simulink library "Cust_Library_planarPKM"  (R2024a)
settings: Solver=VariableStepAuto  StartTime=0.0  StopTime=10.0  RelTol=1e-3
undefined symbols (not defined in the file): param
libraries: simulink x1
(part 2 of 2)

== matlab function Cust_Library_planarPKM/Calculate time derivatives of Jacobian/Calculate_derivative_of_Jacobian_matrices ==
  data: qj_rad input; xEE_ input; dqj_rad input; dxEE_ input; dJinv_hredqax_3RRRreturn output; dJ_hredxqa_3RRRreturn output; dJinv_hqx_3RRRreturn output; l_all parameter; dJacA_hredx_3RRRreturn output; dJacB_hredqa_3RRRreturn output; r_BasisPla_MobPla parameter
function [dJinv_hredqax_3RRRreturn, dJ_hredxqa_3RRRreturn, dJinv_hqx_3RRRreturn, dJacA_hredx_3RRRreturn, dJacB_hredqa_3RRRreturn] ...
    = calcJac(qj_rad, xEE_, dqj_rad, dxEE_, l_all, r_BasisPla_MobPla)
    % Function for determining the time derivatives of the Jacobi matrices based on complete constraints h and reduced constraints hred  
    % Input:
    % qj_rad in rad: Joint coordinates (9x1)
    % dqj_rad in rad: Joint velocities (9x1)
    % xEE_ in m and rad: Platform coordinates in the base CS (3x1)
    % dxEE_ in m and rad: Platform velocities (3x1)
    %
    % Output:
    % dJinv_hqx_3RRRreturn: Time derivative of the Jacobian matrix for projection from ddx to ddq(3x9)
    % dJ_hredxqa_3RRreturn: Temporal derivative of the Jacobian matrix for projection ddqa onto ddx (3x3)
    % dJinv_hredqax_3RRreturn: Temporal derivative of the Jacobian matrix for projection ddx onto ddqa (3x3)
    
    % Aran Mohammad, aran.mohammad@imes.uni-hannover.de, 2022-12
    % (C) Institute for Mechatronic Systems, Leibniz University Hanover
      
      
xEE = [xEE_(1); xEE_(2); 0; 0; 0; xEE_(3)];
dxEE = [dxEE_(1); dxEE_(2); 0; 0; 0; dxEE_(3)];


dJinv_hredqax_3RRRreturn = dJinv_hredqax_3RRR(qj_rad, dqj_rad, xEE, dxEE, l_all, r_BasisPla_MobPla);

dJ_hredxqa_3RRRreturn = dJ_hredxqa_3RRR(qj_rad, dqj_rad, xEE, dxEE, l_all, r_BasisPla_MobPla);

dJinv_hqx_3RRRreturn = transpose(dJinv_hqx_3RRR(qj_rad, dqj_rad, xEE, dxEE, l_all, r_BasisPla_MobPla));

dJacA_hredx_3RRRreturn = dJacA_hredx_3RRR(qj_rad, dqj_rad, xEE, dxEE, l_all, r_BasisPla_MobPla);
dJacB_hredqa_3RRRreturn = dJacB_hredqa_3RRR(qj_rad, dqj_rad, xEE, dxEE, l_all, r_BasisPla_MobPla);

== matlab function Cust_Library_planarPKM/Calculate Jacobian matrices/calculate_Jacobian ==
  data: qj_rad input; xEE_ input; det_JacA_hredx_3RRR output; det_JacB_hredqa_3RRR output; cond_JacA_hredx_3RRR output; cond_JacB_hredqa_3RRR output; JacA_hredx_3RRR output; JacB_hredqa_3RRR output; J_hredxqa_ind_3RRRreturn output; Jinv_hredqax_ind_3RRRreturn output; Jinv_hqx_ind_3RRRreturn output; l_all_id parameter; det_JacA_hredx_ind_3RRRreturn_homogen output; det_JacB_hredqa_ind_3RRRreturn_homogen output; Jinv_hqx_dq_dqa output; cond_Jac_hredxqa_3RRR output; r_fixPlat_j parameter; r_mobPlat_j parameter; beta_j parameter; psi_j parameter
function [det_JacA_hredx_3RRR, det_JacB_hredqa_3RRR, cond_JacA_hredx_3RRR, cond_JacB_hredqa_3RRR, ...
          JacA_hredx_3RRR, JacB_hredqa_3RRR, J_hredxqa_ind_3RRRreturn, Jinv_hredqax_ind_3RRRreturn,...
          Jinv_hqx_ind_3RRRreturn, det_JacA_hredx_ind_3RRRreturn_homogen, det_JacB_hredqa_ind_3RRRreturn_homogen, ...
          Jinv_hqx_dq_dqa, cond_Jac_hredxqa_3RRR] = calcJac(qj_rad, xEE_, l_all_id, r_fixPlat_j, r_mobPlat_j, beta_j, psi_j)
    % Function for determining the Jacobi matrices based on complete constraints h and reduced constraints hred  
    % Input:
    % qj_rad in rad: Joint coordinates (9x1)
    % xEE_ in m and rad: Platform coordinates in the base CS (3x1)
    %
    % Output:
    % JacA_hredx_ind_3RRRreturn: Jacobian matrix of the direct kinematics (3x3)
    % JacB_hredqa_ind_3RRreturn: Jacobian matrix of the inverse kinematics (3x3)
    % Jinv_hqx_ind_3RRreturn: Inverse Jacobian matrix for projection from dx to dq(3x9)
    % J_hredxqa_ind_3RRreturn: Jacobian matrix for projection dqa onto dx (3x3)
    % Jinv_hredqax_ind_3RRreturn: Inverse Jacobian matrix for projection dx onto dqa (3x3)
    % det_JacA_hredx_3RRR: Determinant of the Jacobian matrix of the direct kinematics (1x1)
    % det_JacB_hredqa_3RRR: Determinant of the Jacobian matrix of the inverse kinematics (1x1)
   
    % Aran Mohammad, aran.mohammad@imes.uni-hannover.de, 2022-12
    % (C) Institute for Mechatronic Systems, Leibniz University Hanover
      
xEE = [xEE_(1); xEE_(2); 0; 0; 0; xEE_(3)];

Jinv_hqx_3RRRreturn = zeros(3,3);%transpose(Jinv_hqx_3RRR(qj_rad, xEE, l_all, r_BasisPla_MobPla));
Jinv_hredqax_3RRRreturn = zeros(3,3);%Jinv_hredqax_3RRR(qj_rad, xEE, l_all, r_BasisPla_MobPla);
J_hredxqa_3RRRreturn = zeros(3,3);% J_hredxqa_3RRR(qj_rad, xEE, l_all, r_BasisPla_MobPla);

%% individuelle kinematische Parameter
JacA_hredx_ind_3RRRreturn = JacA_hredx_ind_3RRR(qj_rad, xEE, l_all_id, r_fixPlat_j, r_mobPlat_j, psi_j, beta_j);
JacB_hredqa_ind_3RRRreturn = JacB_hredqa_ind_3RRR(qj_rad, xEE, l_all_id, r_fixPlat_j, r_mobPlat_j, psi_j, beta_j);
Jinv_hqx_ind_3RRRreturn = transpose(Jinv_hqx_ind_3RRR(qj_rad, xEE, l_all_id, r_fixPlat_j, r_mobPlat_j, psi_j, beta_j));

Jinv_hredqax_ind_3RRRreturn = -inv(JacB_hredqa_ind_3RRRreturn)*JacA_hredx_ind_3RRRreturn;
J_hredxqa_ind_3RRRreturn = inv(Jinv_hredqax_ind_3RRRreturn);

Jinv_hqx_dq_dqa = Jinv_hqx_ind_3RRRreturn / Jinv_hredqax_ind_3RRRreturn;

JacA_hredx_3RRR = JacA_hredx_ind_3RRRreturn;
JacB_hredqa_3RRR = JacB_hredqa_ind_3RRRreturn;

% Determinanten
det_JacA_hredx_3RRR = det(JacA_hredx_ind_3RRRreturn);
det_JacB_hredqa_3RRR = det(JacB_hredqa_ind_3RRRreturn);
cond_JacA_hredx_3RRR = cond(JacA_hredx_ind_3RRRreturn,2);
cond_JacB_hredqa_3RRR = cond(JacB_hredqa_ind_3RRRreturn,2);
cond_Jac_hredxqa_3RRR = cond(J_hredxqa_ind_3RRRreturn,2);


JacA_hredx_ind_3RRRreturn_homogen = JacA_hredx_ind_3RRRreturn;
JacA_hredx_ind_3RRRreturn_homogen(:,3) = JacA_hredx_ind_3RRRreturn(:,3)./r_mobPlat_j(1);
JacB_hredqa_ind_3RRRreturn_homogen = JacB_hredqa_ind_3RRRreturn./l_all_id(1);
det_JacA_hredx_ind_3RRRreturn_homogen = det(JacA_hredx_ind_3RRRreturn_homogen);
det_JacB_hredqa_ind_3RRRreturn_homogen = det(JacB_hredqa_ind_3RRRreturn_homogen);

== matlab function Cust_Library_planarPKM/Localize contact point on second link via particle filter/MATLAB Function4 ==
  data: trigger input; Tauext input; predLoc_2D output; predBody input; q input; dq input; x input; dx input; Jinv_hqx_ind input; J_hredxqa input; n_particle input; predForce_2D output; l_all parameter; predLoc_3D output; predForce_3D output; r_BasisPla_MobPla parameter; l_all_id parameter; r_fixPlat_j parameter; r_mobPlat_j parameter; psi_j parameter; x_N_2D parameter; x_CovR_Inv_2D parameter; x_N_3D parameter; x_CovR_Inv_3D parameter; pf_dim parameter
function [predLoc_2D, predForce_2D, predLoc_3D, predForce_3D] = ...
    LocIsol_particleFilter_red_(trigger, Tauext,predBody, q, dq, x, dx, Jinv_hqx_ind, J_hredxqa,...
    n_particle, l_all, r_BasisPla_MobPla, l_all_id, r_fixPlat_j, r_mobPlat_j, psi_j, x_N_2D, x_CovR_Inv_2D, x_N_3D, x_CovR_Inv_3D, pf_dim)
   
    predLoc_2D = 0;
    predForce_2D = 0;
    predLoc_3D = 0;
    predForce_3D = zeros(1,2);
    if pf_dim == 2
        [predLoc_2D, predForce_2D, ~, ~] = LocIsol_particleFilter_red(trigger,Tauext, predBody, q, dq, x, dx, Jinv_hqx_ind, J_hredxqa, ...
            n_particle, l_all, r_BasisPla_MobPla, l_all_id, r_fixPlat_j, r_mobPlat_j, psi_j, x_N_2D, x_CovR_Inv_2D);
    elseif pf_dim == 3
        [predLoc_3D, predForce_3D, ~, ~] = LocIsol_particleFilter(trigger, Tauext, predBody, q, dq, x, dx, Jinv_hqx_ind, J_hredxqa,...
            n_particle, l_all, r_BasisPla_MobPla, l_all_id, r_fixPlat_j, r_mobPlat_j, psi_j, x_N_3D, x_CovR_Inv_3D);
    end
end

== matlab function Cust_Library_planarPKM/Moe_ArMo ==
  data: x_soll input; mode output size=1; x_ist input; qa_ist input; dqa_ist input; dx_soll input; J_hredxqa input; ddx_soll input; dJ_hredxqa input; param parameter; tau_soll output size=[3,1]; MMQa_ist input; dx_ist input; ddqa_prev input; dqa_out output; ddqa_out output; tau_out output; e_qa output size=[3,1]; de_qa output size=[3,1]; qa_soll output size=[3,1]; dqa_prev input size=[3,1]; h_kappa_out output size=1; dq_all output size=[12,1]; ddq_all output size=[12,1]; tau_all output size=[12,1]; mode_prev input; D_pose input; K_pose input; tau_prev input; taucX_ist input; kappa_ist input; min_dist input; sigma_activ_list output; h_kappa_flag_out output; x_soll_r output; dkappa input; dmindist input; J_kappa input; J_dist input; dJ_kappa input; dJ_dist input; MMX_ist input; taucQa_ist input; tauCQa_ist input; xp_soll input; dxp_soll input; ddxp_soll input; xp_KSGj_ist input; dxp_KSGj_ist input; dRxp_ist input; R_0Gj input; dR_0Gj input; J_xpqa input; J_xpqa_KS0 input; dJ_xpqa_KS0 input; dxp_KS0_ist input; xp_KS0_ist input; dJ_xpqa input; predbody input; BP_Retr_calc_run_KSGj input; rr_level input; rueck_KS0 input; lambda_dq input; lambda_ddq input; lambda_tau input; pd_reglerQ input; kappa_mindist_lim input; priority_x input; gain_check_status_kappa input; gain_check_status_mindist input; activate_bp_UNB input; kappa_traj_soll input; mindist_traj_soll input; rueckzug_aktiv input; reaction_angle_rad input; x_ist_r output; dq_Jkappa output; dq_Jdist output; mode_nan output; clamping_predicted input; clampingBody_predicted input; clampingreaction_aktiv input; traj_qap_soll_cl input; J_q_qa input; dJ_q_qa input; M_kappa output; M_dist output; q_ist_rad input; dq_ist_rads input
function [mode, tau_soll, dqa_out, ddqa_out, tau_out, e_qa, de_qa, qa_soll,...
          h_kappa_out, dq_all,  ddq_all, tau_all, sigma_activ_list, h_kappa_flag_out, ...
          x_soll_r, x_ist_r, dq_Jkappa, dq_Jdist, mode_nan, M_kappa, M_dist] = ...
            fcn(x_soll, x_ist, qa_ist, dqa_ist, dx_soll, J_hredxqa, ddx_soll, ...
                dJ_hredxqa, param, MMQa_ist, dx_ist, ddqa_prev, dqa_prev, mode_prev, ...
                D_pose, K_pose, tau_prev, taucX_ist, kappa_ist, min_dist, dkappa, ...
                dmindist, J_kappa, J_dist, dJ_kappa, dJ_dist, MMX_ist, taucQa_ist, ...
                tauCQa_ist, xp_soll, dxp_soll, ddxp_soll, xp_KSGj_ist, dxp_KSGj_ist, dRxp_ist, ...
                R_0Gj, dR_0Gj, J_xpqa, J_xpqa_KS0, dJ_xpqa_KS0, dxp_KS0_ist, xp_KS0_ist, ...
                dJ_xpqa, predbody, BP_Retr_calc_run_KSGj, rr_level, rueck_KS0, ...
                lambda_dq, lambda_ddq, lambda_tau, pd_reglerQ, kappa_mindist_lim, priority_x,   gain_check_status_kappa, gain_check_status_mindist,...
                activate_bp_UNB, kappa_traj_soll, mindist_traj_soll, rueckzug_aktiv, reaction_angle_rad,...
                clamping_predicted, clampingBody_predicted, clampingreaction_aktiv, traj_qap_soll_cl, J_q_qa, dJ_q_qa, q_ist_rad, dq_ist_rads)
            

       mode = zeros(1,1);
       tau_soll = zeros(3,1);
       dqa_out = zeros(3,1);
       ddqa_out = zeros(3,1);
       tau_out = zeros(3,1);
       e_qa = zeros(3,1);
       de_qa = zeros(3,1);
       qa_soll = zeros(3,1);
       h_kappa_out = zeros(1,1);
       dq_all = zeros(12,1);
       ddq_all = zeros(12,1);
       tau_all = zeros(12,1);
       sigma_activ_list = zeros(8,1);
       h_kappa_flag_out = zeros(1,1);
       x_soll_r = zeros(3,1);
       x_ist_r = zeros(3,1);
       dq_Jkappa = zeros(4,1);
       dq_Jdist  = zeros(4,1);
       mode_nan = 0;
       M_kappa = nan;
       M_dist = nan;
    if rr_level ~= 0 %&& rueckzug_aktiv
        [mode, tau_soll, dqa_out, ddqa_out, tau_out, e_qa, de_qa, qa_soll,...
          h_kappa_out, dq_all,  ddq_all, tau_all, sigma_activ_list, h_kappa_flag_out, ...
          x_soll_r, x_ist_r, dq_Jkappa, dq_Jdist, mode_nan, M_kappa, M_dist] = ...
        calc_rr(x_soll, x_ist, qa_ist, dqa_ist, dx_soll, J_hredxqa, ddx_soll, ...
                    dJ_hredxqa, param, MMQa_ist, dx_ist, ddqa_prev, dqa_prev, mode_prev, ...
                    D_pose, K_pose, tau_prev, taucX_ist, kappa_ist, min_dist, dkappa, ...
                    dmindist, J_kappa, J_dist, dJ_kappa, dJ_dist, MMX_ist, taucQa_ist, ...
                    tauCQa_ist, xp_soll, dxp_soll, ddxp_soll, xp_KSGj_ist, dxp_KSGj_ist, dRxp_ist, ...
                    R_0Gj, dR_0Gj, J_xpqa, J_xpqa_KS0, dJ_xpqa_KS0, dxp_KS0_ist, xp_KS0_ist, ...
                    dJ_xpqa, predbody, BP_Retr_calc_run_KSGj, rr_level, rueck_KS0, ...
                    lambda_dq, lambda_ddq, lambda_tau, pd_reglerQ, kappa_mindist_lim, priority_x,   gain_check_status_kappa, gain_check_status_mindist,...
                    activate_bp_UNB, kappa_traj_soll, mindist_traj_soll, rueckzug_aktiv, reaction_angle_rad,...
                    clamping_predicted, clampingBody_predicted, clampingreaction_aktiv, traj_qap_soll_cl, J_q_qa, dJ_q_qa, q_ist_rad, dq_ist_rads);

    else 
       mode = zeros(1,1);
       tau_soll = zeros(3,1);
       dqa_out = zeros(3,1);
       ddqa_out = zeros(3,1);
       tau_out = zeros(3,1);
       e_qa = zeros(3,1);
       de_qa = zeros(3,1);
       qa_soll = zeros(3,1);
       h_kappa_out = zeros(1,1);
       dq_all = zeros(12,1);
       ddq_all = zeros(12,1);
       tau_all = zeros(12,1);
       sigma_activ_list = zeros(8,1);
       h_kappa_flag_out = zeros(1,1);
       x_soll_r = zeros(3,1);
       x_ist_r = zeros(3,1);
       dq_Jkappa = zeros(4,1);
       dq_Jdist  = zeros(4,1);
       mode_nan = 0;
       M_kappa = nan;
       M_dist = nan;
    end

== stateflow chart Cust_Library_planarPKM/Statemachine ==
  state State0 %Eingang, warte auf kommunikation mit den Motoren
    entry:
    control 		= 4;%Ist-Winkel in die BP
    bp_on 		= 0;%BP unbenutzt
    bp_retr_on       = 0;% BP für Retr unbenutzt
    tr_on 		      = 0;%Traj unbenutzt
    gmt_on            = 0;%GMT unbenutzt
    error 			= 0;%Motor kann starten
    control_out      = 0;%Ist-Werte als Soll-Werte
    state = 0;
  state State1 %Kommunikation funktioniert
    entry:
    control 		= 4;%Ist-Winkel in die BP
    bp_on 		= 0;%BP unbenutzt
    bp_retr_on       = 0;% BP für Retr unbenutzt
    tr_on 		      = 0;%Traj unbenutzt
    gmt_on            = 0;%GMT unbenutzt
    error 			= 0;%Motor kann starten
    control_out      = 0;%Ist-Werte als Soll-Werte
    state = 1;
  state Home Position Drive [group]
    state State7 %Setzte Vorgaben, Überprüfe ob
      %Zielpunkt valid ist
      entry:
      control 		 	= 2;%Home-Winkel in die BP
      bp_on 			= 0; %BP unbenutzt
      bp_retr_on       = 0;% BP für Retr unbenutzt
      tr_on 		      = 0;%Traj unbenutzt
      gmt_on            = 0;%GMT unbenutzt
      error 			= 0;%Motor bleibt an
      control_out      = 1;%BP-Werte als Soll-Werte
      state = 7;
    state State8 %Starte Bahnplanung
      entry:
      control 		 	= 2;%Ziel-Winkel in die BP
      bp_on 			= 1; %BP wird genutzt
      bp_retr_on       = 0;% BP für Retr unbenutzt
      tr_on 		      = 0;%Traj unbenutzt
      gmt_on            = 0;%GMT unbenutzt
      error 			= 0;%Motor bleibt an
      control_out      = 1;%BP-Werte als Soll-Werte
      state = 8;
    state State9 %Starte Bahnplanung
      entry:
      control 		 	= 2;%Ziel-Winkel in die BP
      bp_on 			= 0; %BP beendet
      bp_retr_on       = 0;% BP für Retr unbenutzt
      tr_on 		      = 0;%Traj unbenutzt
      gmt_on            = 0;%GMT unbenutzt
      error 			= 0;%Motor bleibt an
      control_out      = 1;%BP-Werte als Soll-Werte
      state = 9;
    State7 %Setzte Vorgaben, Überprüfe ob -> State8 %Starte Bahnplanung [order 1] : [bp_valid ==1]
    State8 %Starte Bahnplanung -> State9 %Starte Bahnplanung [order 2] : [bp_calc_run == 0]
  state Trajectory Drive [group]
    state State10 %Setzte Vorgaben, Überprüfe ob
      %Zielpunkt valid ist
      entry:
      control 		 	= 3;%Startwinkel der traj in BP
      bp_on 			= 0;%BP unbenutzt
      bp_retr_on       = 0;% BP für Retr unbenutzt
      tr_on 			= 0;%Traj unbenutzt
      gmt_on            = 0;%GMT unbenutzt
      error 			= 0;%Motor bleibt an
      control_out      = 1;%BP-Werte als Soll-Werte
      state = 10;
    state State11 %Fahre zum Ausgangspunkt
      entry:
      control 		 	= 3;%Startwinkel der traj in BP
      bp_on 			= 1;%BP wird genutzt
      bp_retr_on       = 0;% BP für Retr unbenutzt
      tr_on 			= 0;%Traj unbenutzt
      gmt_on            = 0;%GMT unbenutzt
      error 			= 0;%Motor bleibt an
      control_out      = 1;%BP-Werte als Soll-Werte
      state = 11;
    state State12 %Validiere Trajektorie und setze Vorgaben
      entry:
      control 		 	= 4;%Ist-Winkel in die BP
      bp_on 			= 0;%BP unbenutzt
      bp_retr_on       = 0;% BP für Retr unbenutzt
      tr_on 			= 0;%Traj unbenutzt
      gmt_on            = 0;%GMT unbenutzt
      error 			= 0;%Motor bleibt an
      control_out      = 1;%BP-Werte als Soll-Werte
      state = 12;
    state State13 %Starte Trajektorie
      entry:
      control 		 	= 4;%Ist-Winkel in die BP
      bp_on 			= 0;%BP unbenutzt
      bp_retr_on       = 0;% BP für Retr unbenutzt
      tr_on 		      = 1;%Traj wird genutzt
      gmt_on            = 0;%GMT unbenutzt
      error 			= 0;%Motor bleibt an
      control_out      = 2;%Traj-Werte als Soll-Werte
      state = 13;
    state State14 %Starte Trajektorie
      entry:
      control 		 	= 4;%Ist-Winkel in die BP
      bp_on 			= 0;%BP unbenutzt
      bp_retr_on       = 0;% BP für Retr unbenutzt
      tr_on 		      = 0;%Traj unbenutzt
      gmt_on            = 0;%GMT unbenutzt
      error 			= 0;%Motor bleibt an
      control_out      = 2;%Traj-Werte als Soll-Werte
      state = 14;
    State10 %Setzte Vorgaben, Überprüfe ob -> State11 %Fahre zum Ausgangspunkt [order 1] : [bp_valid ==1]
    State11 %Fahre zum Ausgangspunkt -> State12 %Validiere Trajektorie und setze Vorgaben [order 1] : [bp_calc_run ==0  & tr_in_starting_pos == 1]
    State12 %Validiere Trajektorie und setze Vorgaben -> State13 %Starte Trajektorie [order 1] : [tr_valid == 1]
    State13 %Starte Trajektorie -> State14 %Starte Trajektorie [order 2] : [tr_calc_run ==0]
  state Target Position Drive [group]
    state State2 %Setzte Vorgaben, Überprüfe ob
      %Zielpunkt valid ist
      entry:
      control 			= 1;%Ziel-Winkel in die BP
      bp_on 			= 0; %BP unbenutzt
      bp_retr_on       = 0;% BP für Retr unbenutzt
      tr_on 		      = 0;%Traj unbenutzt
      gmt_on            = 0;%GMT unbenutzt
      error 			= 0;%Motor bleibt an
      control_out      = 1;%BP-Werte als Soll-Werte
      state = 2;
    state State3 %Starte Bahnplanung
      entry:
      control 			= 1;%Ziel-Winkel in die BP
      bp_on 			= 1; %BP wird genutzt
      bp_retr_on       = 0;% BP für Retr unbenutzt
      tr_on 		      = 0;%Traj unbenutzt
      gmt_on            = 0;%GMT unbenutzt
      error 			= 0;%Motor bleibt an
      control_out      = 1;%BP-Werte als Soll-Werte
      state = 3;
    state State4 %Starte Bahnplanung
      entry:
      control 			= 1;%Ziel-Winkel in die BP
      bp_on 			= 0; %BP beendet
      bp_retr_on       = 0;% BP für Retr unbenutzt
      tr_on 		      = 0;%Traj unbenutzt
      gmt_on            = 0;%GMT unbenutzt
      error 			= 0;%Motor bleibt an
      control_out      = 1;%BP-Werte als Soll-Werte
      state = 4;
    State2 %Setzte Vorgaben, Überprüfe ob -> State3 %Starte Bahnplanung [order 1] : [bp_valid ==1]
    State3 %Starte Bahnplanung -> State4 %Starte Bahnplanung [order 1] : [bp_calc_run == 0]
  state Geomagic Touch [group]
    state State15
      entry:
      control 		 	= 2;%Startwinkel der traj in BP
      bp_on 			= 0;%BP unbenutzt
      bp_retr_on       = 0;% BP für Retr unbenutzt
      tr_on 			= 0;%Traj unbenutzt
      gmt_on            = 1;%GMT benutzt
      error 			= 0;%Motor bleibt an
      control_out      = 3;%GMT-Werte als Soll-Werte
      state = 15;
  state Retraction Drive [group]
    state State25 %Setzte Vorgaben, Überprüfe ob
      %Zielpunkt valid ist
      entry:
      control 			= 5;%Ziel-Winkel in die BP
      bp_on 			= 1; %BP unbenutzt
      bp_retr_on       = 0;% BP für Retr unbenutzt
      tr_on 		      = 0;%Traj unbenutzt
      gmt_on            = 0;%GMT unbenutzt
      error 			= 0;%Motor bleibt an
      control_out      = 1;%BP-Werte als Soll-Werte
      state = 25;
    state State26 %Starte Bahnplanung
      entry:
      control 			= 5;%Ziel-Winkel in die BP
      bp_on 			= 1; %BP unbenutzt
      bp_retr_on       = 1;% BP für Retr wird benutzt
      tr_on 		      = 0;%Traj unbenutzt
      gmt_on            = 0;%GMT unbenutzt
      error 			= 0;%Motor bleibt an
      control_out      = 4;%BP-Werte als Soll-Werte
      state = 26;
    state State27 %Starte Bahnplanung
      entry:
      control 			= 5;%Ziel-Winkel in die BP
      bp_on 			= 0; %BP unbenutzt
      bp_retr_on       = 0;% BP für Retr wird benutzt
      tr_on 		      = 0;%Traj unbenutzt
      gmt_on            = 0;%GMT unbenutzt
      error 			= 0;%Motor bleibt an
      control_out      = 4;%BP-Werte als Soll-Werte
      state = 27;
    State25 %Setzte Vorgaben, Überprüfe ob -> State26 %Starte Bahnplanung : [Init_Retr_valid==1]
    State26 %Starte Bahnplanung -> State27 %Starte Bahnplanung [order 1] : [BP_Retr_calc_run == 0]
  state Error_Case2 : Zielgrößen der Trajektorien liegen nicht im [group]
    Arbeitsraum
    state State998
      entry:
      control 		= 4;%Ist-Winkel in die BP
      bp_on 		= 0;%BP ungenutzt
      bp_retr_on       = 0;% BP für Retr unbenutzt
      tr_on 		      = 0;%Traj ungenutzt
      gmt_on            = 0;%GMT unbenutzt
      error 			= 1;%
      control_out      = 0;%Ist-Werte als Soll-Werte
      state = 21;
  state Error_Case1 : Arbeitsraumgrenzen Erreicht [group]
    state State999
      entry:
      control 		= 4;%Ist-Winkel in die BP
      bp_on 		= 0;%BP ungenutzt
      bp_retr_on       = 0;% BP für Retr unbenutzt
      tr_on 		      = 0;%Traj ungenutzt
      gmt_on            = 0;%GMT unbenutzt
      error 			= 1;%Motor Aus
      control_out      = 0;%Ist-Werte als Soll-Werte
      state = 20;
    note: Error Case : Winkel weit unterhalb des validen Bereiches
        |
        | Wartet auf
        | -Bis keine BP mehr durchgeführt wird
        | -Anweisung zum Anfahren der Home Position
  (default) -> State0 %Eingang, warte auf kommunikation mit den Motoren
  State0 %Eingang, warte auf kommunikation mit den Motoren -> State999 [order 2] : [run_overflow ==0  | reset ==1 ]
  State0 %Eingang, warte auf kommunikation mit den Motoren -> State1 %Kommunikation funktioniert [order 1] : [GUI_started == 1 ]
  State14 %Starte Trajektorie -> State1 %Kommunikation funktioniert [order 1] : [trajectory_run == 0]
  State998 -> State1 %Kommunikation funktioniert : [Enable_Drive == 1]
  State1 %Kommunikation funktioniert -> State999 [order 3] : [run_overflow ==0  | reset ==1 ]
  State27 %Starte Bahnplanung -> State1 %Kommunikation funktioniert [order 2] : [ target_run == 0]
  State11 %Fahre zum Ausgangspunkt -> State1 %Kommunikation funktioniert [order 3] : [trajectory_run == 0]
  State999 -> State1 %Kommunikation funktioniert : [Enable_Drive == 1]
  State1 %Kommunikation funktioniert -> State15 [order 5] : [gmt_act==1&tr_calc_run == 0 & bp_calc_run ==0 & controlword==15]
  State10 %Setzte Vorgaben, Überprüfe ob -> State1 %Kommunikation funktioniert [order 2] : [reset == 1]
  State4 %Starte Bahnplanung -> State1 %Kommunikation funktioniert [order 2] : [ target_run == 0]
  State15 -> State1 %Kommunikation funktioniert [order 2] : [gmt_act==0]
  State2 %Setzte Vorgaben, Überprüfe ob -> State1 %Kommunikation funktioniert [order 2] : [bp_valid ==0 | reset == 1 ]
  State1 %Kommunikation funktioniert -> State10 %Setzte Vorgaben, Überprüfe ob [order 4] : [tr_calc_run == 0 & bp_calc_run ==0 & trajectory_run_trig ==1 & controlword == 15]
  State1 %Kommunikation funktioniert -> State2 %Setzte Vorgaben, Überprüfe ob [order 2] : [tr_calc_run == 0 & bp_calc_run ==0 & target_run_trig ==1 & controlword == 15 ]
  State9 %Starte Bahnplanung -> State1 %Kommunikation funktioniert [order 2] : [home_run == 0]
  State7 %Setzte Vorgaben, Überprüfe ob -> State1 %Kommunikation funktioniert [order 2] : [bp_valid ==0 | reset == 1 ]
  State1 %Kommunikation funktioniert -> State7 %Setzte Vorgaben, Überprüfe ob [order 1] : [tr_calc_run == 0 & bp_calc_run ==0 & home_run_trig ==1 & controlword == 15]
  State3 %Starte Bahnplanung -> State25 %Setzte Vorgaben, Überprüfe ob [order 3] : [Init_retr==1 & run_overflow==1 | (target_run == 0 & bp_calc_run ==1)]
  State15 -> State999 [order 1] : [gmt_valid==0]
  State10 %Setzte Vorgaben, Überprüfe ob -> State998 [order 3] : [bp_valid ==0 ]
  State12 %Validiere Trajektorie und setze Vorgaben -> State998 [order 2] : [tr_valid ==0  | reset ==1]
  State13 %Starte Trajektorie -> State998 [order 1] : [tr_valid ==0 ]
  State8 %Starte Bahnplanung -> State999 [order 1] : [run_overflow ==0  | reset ==1  | (home_run == 0 & bp_calc_run ==1)]
  State11 %Fahre zum Ausgangspunkt -> State999 [order 2] : [run_overflow ==0 | reset ==1  | (trajectory_run == 0 & bp_calc_run ==1)]
  State3 %Starte Bahnplanung -> State999 [order 2] : [run_overflow ==0  | reset ==1  | (target_run == 0 & bp_calc_run ==1)]
  State26 %Starte Bahnplanung -> State999 [order 2] : [run_overflow ==0  | reset ==1  | (target_run == 0 & BP_Retr_calc_run ==1)]
  State9 %Starte Bahnplanung -> State999 [order 1] : [run_overflow ==0  | reset ==1]
  State4 %Starte Bahnplanung -> State999 [order 1] : [run_overflow ==0  | reset ==1]
  State27 %Starte Bahnplanung -> State999 [order 1] : [run_overflow ==0  | reset ==1]
  State13 %Starte Trajektorie -> State999 [order 3] : [run_overflow ==0  | reset ==1 | (trajectory_run == 0 & tr_calc_run ==1)]
  State14 %Starte Trajektorie -> State999 [order 2] : [run_overflow ==0  | reset ==1]
  data: tr_valid input; bp_valid input; target_run input; target_run_trig input; bp_on output; reset input; GUI_started input; bp_calc_run input; controlword input; home_run_trig input; home_run input; error output; control output; control_out output; run_overflow input; Enable_Drive input; trajectory_run_trig input; trajectory_run input; gmt_act input; gmt_valid input; Init_retr input; tr_calc_run input; Init_Retr_valid input; BP_Retr_calc_run input; tr_on output; tr_in_starting_pos input; state output; gmt_on output; bp_retr_on output

== matlab function Cust_Library_planarPKM/Localize collided body/Localize collided body ==
  data: predprob_all output; predprob output; pred_body_ffnn output; Contact_detected input; Fext_obs input; Tauext_qa input; distances input; angles input; pred_body output; min_dist_threshold parameter; min_angle_threshold_deg parameter; min_torque_threshold parameter; ffnn_ClCollB_param parameter
function [predprob_all, predprob, pred_body_ffnn, pred_body] = localize_chain_link(Contact_detected, Fext_obs, Tauext_qa, distances, angles, ...
        min_dist_threshold, min_angle_threshold_deg, min_torque_threshold, ffnn_ClCollB_param)
    if Contact_detected
        pred_body = localize_chain_link_thresholddecision(Tauext_qa, distances, angles, min_dist_threshold, min_angle_threshold_deg, min_torque_threshold);
        [predprob_all,pred_body_ffnn] = localize_chain_link_FFNN(Fext_obs,Tauext_qa, ffnn_ClCollB_param, distances, angles);
        predprob = predprob_all(pred_body_ffnn); 
    else
        predprob_all = zeros(7,1);
        predprob = 0;
        pred_body=0;
        pred_body_ffnn = 0;        
    end

== matlab function Cust_Library_planarPKM/Calculate_dynamics_terms/MATLAB Function ==
  data: qj_rad input; cvecred_X output; dqj_rad input; xEE input; dxEE input; J_hredxqa input; Jinv_hredqax input; dJ_hredxqa input; Fext input; tauQa input; Cred_X output; Mred_X output; tauFrared_X output; Mred_Qa output; MDP parameter; cvecred_Qa output; Cred_Qa output; ddx output; ddqa output; l_all parameter; r_BasisPla_MobPla parameter
function [cvecred_X,Cred_X,Mred_X,tauFrared_X,Mred_Qa, cvecred_Qa, Cred_Qa, ddx, ddqa] = fcn(qj_rad, dqj_rad, xEE, dxEE, J_hredxqa, Jinv_hredqax, dJ_hredxqa, Fext, tauQa,...
    MDP, l_all, r_BasisPla_MobPla)
    % Function for determining the dynamic terms
    % Input:
    % qj_rad in rad: Joint coordinates (9x1)
    % dqj_rad in rad/s: Joint velocities (9x1)
    % xEE in m and rad: Platform coordinates in the base CS (6x1)
    % dxEE in/s m and rad/s: Platform velocities in the base CS (6x1)
    % J_hredxqa: Jacobian matrix to project dqa onto dx (3x3)
    %
    % Output:
    % cvecred_X: Vector of centrifugal and coriolis terms in platform coordinates (3x1)
    % Cred_X: Matrix of centrifugal and coriolis terms in platform coordinates (3x3)
    % Mred_X: Matrix of inertia effects in platform coordinates (3x3)
    % tauFrared_X: Vector of friction effects of the active joints in platform coordinates (3x1)
    % Mred_Qa: Matrix of inertia effects in drive coordinates (3x3)
    
    
    % Aran Mohammad, aran.mohammad@imes.uni-hannover.de, 2022-12
    % (C) Institute for Mechatronic Systems, Leibniz University Hanover

    cvecred_X = transpose(cvecred_mdp_3RRR(qj_rad, dqj_rad, xEE, dxEE, MDP, l_all, r_BasisPla_MobPla));
    Cred_X = Cred_mdp_3RRR(qj_rad, dqj_rad, xEE, dxEE, MDP, l_all, r_BasisPla_MobPla);
    Mred_X = Mred_mdp_3RRR(qj_rad, xEE, MDP, l_all, r_BasisPla_MobPla);
    tauFrared_X = transpose(tauFrared_mdp_3RRR(qj_rad, dqj_rad, xEE, dxEE, MDP, l_all, r_BasisPla_MobPla));
    Mred_Qa = J_hredxqa' * Mred_X * J_hredxqa;
    cvecred_Qa = J_hredxqa'*cvecred_X + Mred_Qa*Jinv_hredqax*dJ_hredxqa*dqj_rad([1 4 7]);
    Cred_Qa = J_hredxqa'*Cred_X*J_hredxqa + Mred_Qa*Jinv_hredqax*dJ_hredxqa;
    
    ddx = Mred_X\ (Jinv_hredqax'*tauQa + cvecred_X + tauFrared_X + Fext);
    ddqa = Mred_Qa\ (tauQa + cvecred_Qa + J_hredxqa'*tauFrared_X + J_hredxqa'*Fext);

== matlab function Cust_Library_planarPKM/LowPF/MATLAB Function16 ==
  data: u_raw input; u_filt output; u_prev input; a input; y_prev input; not_defined_nan output
function  [u_filt, not_defined_nan] = TP1_DiffEq(u_raw, u_prev, a, y_prev)
if isnan(sum(sum(u_raw))) || isinf(sum(sum(u_raw)))
    u_filt = zeros(size(u_raw));
    not_defined_nan = 1;
elseif isnan(sum(sum(TP1_DiffEq(u_raw, u_prev, a, y_prev)))) || isinf(sum(sum(TP1_DiffEq(u_raw, u_prev, a, y_prev))))
        u_filt = zeros(size(u_raw));
        not_defined_nan = 2;
else
    u_filt = TP1_DiffEq(u_raw, u_prev, a, y_prev);
    not_defined_nan = 0;
end

== matlab function Cust_Library_planarPKM/calc_q_rotConstraints/calc_q_rotConstraints ==
  data: qa input; q output; qp input; xEE input; psi_j parameter
function q  = fcn(qa, qp, xEE, psi_j)
phie = xEE(3); 
q13 = phie - (psi_j(1) + qa(1) + qp(1)); 
q23 = phie - (psi_j(2) + qa(2) + qp(2)); 
q33 = phie - (psi_j(3) + qa(3) + qp(3)); 

q = [qa(1); qp(1); q13; ...
    qa(2); qp(2); q23; ...
    qa(3); qp(3); q33];

== matlab function Cust_Library_planarPKM/Classify contact type and clamping chain/MATLAB Function7 ==
  data: bincl_predprob_max output; bincl_predcontact output; bincl_predprob output; Contact_detected input; Fext_obs input; distances input; tauext_obs input; ffnn_clamping_param parameter; mulcl_predprob_chains output; mulcl_predchain output; mulcl_predprob_clampingchain output; ffnn_clamping_chain_param parameter
function [bincl_predprob_max, bincl_predcontact, bincl_predprob, ...
          mulcl_predprob_chains, mulcl_predchain, mulcl_predprob_clampingchain] = ...
         clamping_classification(Contact_detected, Fext_obs, distances, tauext_obs, ffnn_clamping_param, ffnn_clamping_chain_param)
    if Contact_detected
        [bincl_predprob_max, bincl_predcontact, bincl_predprob] = clamping_FFNN(Fext_obs, ffnn_clamping_param);
        [mulcl_predprob_chains,mulcl_predchain] = clamping_chain_FFNN(Fext_obs, ffnn_clamping_chain_param, distances);
        [~, mulcl_predchain] = max(abs(tauext_obs));
        mulcl_predprob_clampingchain = mulcl_predprob_chains(mulcl_predchain); 
    else
        bincl_predprob_max = 0;
        bincl_predcontact = -1;
        bincl_predprob = zeros(1,2);
        
        mulcl_predprob_chains = zeros(3,1);
        mulcl_predchain = 1;
        mulcl_predprob_clampingchain = 0;
    end
